simulink model "subwaycontrolsystem"  (R2012b)
settings: Solver=ode15s  StartTime=0.0  StopTime=2500  MaxStep=0.1  RelTol=1e-6
settings Model: Creator=fanghuixing  LastModifiedBy=fofo
settings SolverCC: MaxConsecutiveZCs=2000  ZeroCrossControl=DisableAll
settings DataIOCC: SignalLoggingSaveFormat=ModelDataLogs  InspectSignalLogs=on
settings OptimizationCC: EfficientMapNaN2IntZero=off
settings DebuggingCC: FcnCallInpInsideContextMsg=UseLocalSettings
settings HardwareCC: TargetIntDivRoundTo=Zero  TargetEndianess=LittleEndian  TargetHWDeviceType=MATLAB Host  ProdEqTarget=off
settings RTWCC: SystemTargetFile=accel.tlc  TemplateMakefile=accel_default_tmf  RTWVerbose=off  ProcessScript=accel_make_rtw_hook
settings CodeAppCC: MaxIdLength=128
settings STFCustomTargetCC: CodeReplacementLibrary=ANSI_C  ConcurrentExecutionCompliant=on  GeneratePreprocessorConditionals=Disable all  SystemTargetFile=accel.tlc

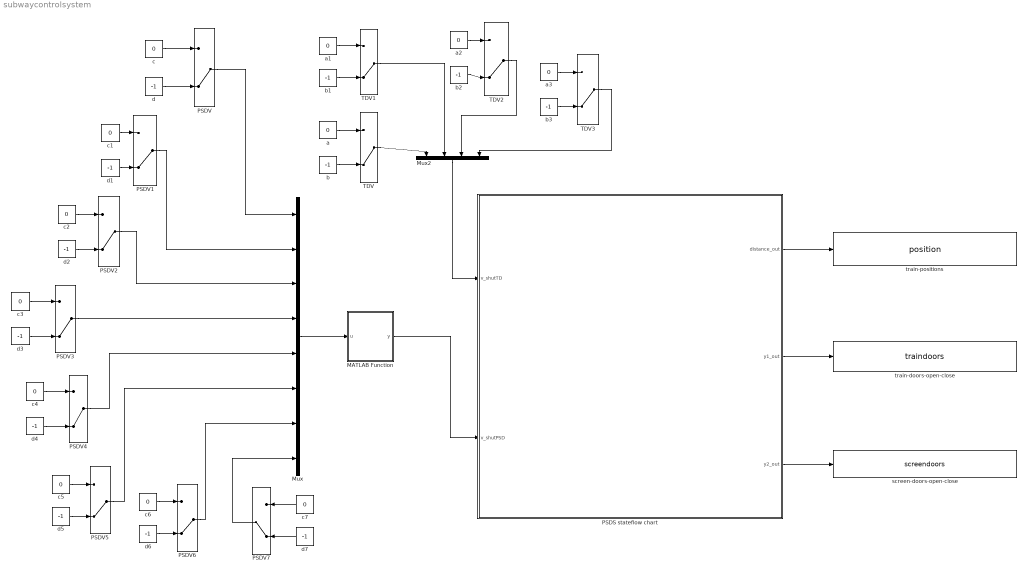
== system subwaycontrolsystem ==
  MATLAB Function : MATLAB Function  TreatAsAtomicUnit=on
  Mux : Mux  Inputs=8
  Mux2 : Mux
  PSDS stateflow chart : Stateflow chart  RequirementInfo="{}  %GIDa_87fe0a43_5411_4934_b3a9_58160d32c6a6"  TreatAsAtomicUnit=on
  PSDV{,1..7} (8 alike) : ManualSwitch  CurrentSetting=0
  TDV{,1..3} (4 alike) : ManualSwitch  CurrentSetting=0
  a{,1..3} (4 alike) : Constant  Value=0
  b{,1..3} (4 alike) : Constant  Value=-1
  c{,1..7} (8 alike) : Constant  Value=0
  "d   " : Constant  Value=-1
  d{1..7} (7 alike) : Constant  Value=-1
  screen-doors-open-close : ToWorkspace  VariableName=screendoors  SampleTime=-1  SaveFormat=Timeseries
  train-doors-open-close : ToWorkspace  VariableName=traindoors  SampleTime=-1  SaveFormat=Structure With Time
  train-positions : ToWorkspace  VariableName=position  SampleTime=-1  SaveFormat=Timeseries
  wires:
  a/1 -> TDV/1
  b/1 -> TDV/2
  TDV/1 -> Mux2/1
  c/1 -> PSDV/1
  "d   "/1 -> PSDV/2
  c1/1 -> PSDV1/1
  d1/1 -> PSDV1/2
  c2/1 -> PSDV2/1
  d2/1 -> PSDV2/2
  c3/1 -> PSDV3/1
  d3/1 -> PSDV3/2
  c4/1 -> PSDV4/1
  d4/1 -> PSDV4/2
  c5/1 -> PSDV5/1
  d5/1 -> PSDV5/2
  c6/1 -> PSDV6/1
  d6/1 -> PSDV6/2
  c7/1 -> PSDV7/1
  d7/1 -> PSDV7/2
  Mux2/1 -> PSDS stateflow chart/1(v_shutTD)
  a1/1 -> TDV1/1
  b1/1 -> TDV1/2
  TDV1/1 -> Mux2/2
  a2/1 -> TDV2/1
  b2/1 -> TDV2/2
  TDV2/1 -> Mux2/3
  a3/1 -> TDV3/1
  b3/1 -> TDV3/2
  TDV3/1 -> Mux2/4
  PSDV/1 -> Mux/1
  PSDV1/1 -> Mux/2
  PSDV2/1 -> Mux/3
  PSDV3/1 -> Mux/4
  PSDV4/1 -> Mux/5
  PSDV5/1 -> Mux/6
  Mux/1 -> MATLAB Function/1(u)
  PSDV6/1 -> Mux/7
  PSDV7/1 -> Mux/8
  MATLAB Function/1(y) -> PSDS stateflow chart/2(v_shutPSD)
  PSDS stateflow chart/2(y1_out) -> train-doors-open-close/1
  PSDS stateflow chart/3(y2_out) -> screen-doors-open-close/1
  PSDS stateflow chart/1(distance_out) -> train-positions/1

== stateflow chart subwaycontrolsystem/PSDS stateflow chart ==
  settings: updateMethod=CONTINUOUS
  state UrgentController [parallel]
    settings: executionOrder=14
    state tmp
      en:t=0;
      du:t_dot=0.5;
    state Delay
      en:t=0;
      du:t_dot=1;
    state D1
      en:t=0;
      du:t_dot=0.5;
    (default) -> Delay
    (junction 1294) -> UrgentController.tmp : {stopDecision(i);}
    UrgentController.tmp -> D1 : [t>=0]
        | {CalDistance(),
        | i=i+1;}
    Delay -> D1 : [t>=150]
        | {i=0;}
    D1 -> (junction 1294) [order 1] : [i!=N&&t>=0]
    D1 -> D1 [order 2] : [i==N&&t>=1]{i=0}
  state Controller1 [parallel]
    settings: executionOrder=16
    state about_to_close2
      en:z=0;
      du:z_dot=1;
    state start
      en:z=0;
      du:z_dot=1;
    state about_to_open2
      en:z=0;
      stop[i]=0;
      du:z_dot=1;
    state idle
      en:z=0;
      du:z_dot=1;
    state about_to_open1
      en:z=0;
      du:z_dot=1;
    state about_to_close1
      en:z=0;
      du:z_dot=1;
    state open1
      en:z=0;
      du:z_dot=1;
    state ring
      du:z_dot=1;
    Controller1.start -> Controller1.start [order 2] : [PSDClosed[stationid][side]==0]
    Controller1.about_to_close2 -> Controller1.about_to_close2 [order 1] : [in(Train1_door.closed)==0]
    (default) -> Controller1.idle
    Controller1.about_to_close1 -> Controller1.about_to_close2 : [z>=5]{closeTD[i]=1;}
    Controller1.about_to_close2 -> Controller1.start [order 2] : [z>=5]
        | {closePSD[stationid][side]=1;}
    Controller1.idle -> Controller1.about_to_open2 [order 1] : [stop[i]==1]
        | {i=1,stationid=Train1.j,
        | side=(dir[i]+1)/2}
    Controller1.start -> Controller1.idle [order 1] : [z>=5]{start[i]=1;}
    Controller1.idle -> Controller1.idle [order 2] : [z>=1&&stop[i]!=1]
        | {position[i]=Train1.distance}
    Controller1.about_to_open2 -> Controller1.about_to_open1 : [z>=5]{openPSD[stationid][side]=1;}
    Controller1.open1 -> Controller1.ring : [z>=10]
    Controller1.about_to_open1 -> Controller1.open1 : [z>=1]{openTD[i]=1;}
    Controller1.ring -> Controller1.about_to_close1 : [z>=20&&z<=30]
  state Train0 [parallel]
    settings: executionOrder=19
    state urgent_inc
      en:urstart[i]=0;
      du:
      distance_dot=dir[i]*v;
      v_dot=0.5;
      distance_out[i]=distance;
    state recover
      du:distance_dot=dir[i]*v;
      v_dot=-0.5;
      distance_out[i]=distance;
    state select
    state urgent_stop
      du:distance_dot=0;
      v_dot=0;distance_out[i]=distance;
      ex:maxv=sqrt(0.5*abs(S[j]-distance))
    state init
      du:time_dot=1;
    state near
      du:
      distance_dot=dir[i]*v;
      v_dot=acc;
      distance_out[i]=distance;
    state urgent_dec
      du:
      distance_dot=dir[i]*v;
      v_dot=-1.5;
      distance_out[i]=distance;
    state stop
      en:v=0;
    state tmp
    state stablerun
      du:
      distance_dot=dir[i]*v;
      v_dot=0;
      distance_out[i]=distance;
    state run
      du:distance_dot=dir[i]*v;
      v_dot=0.5;
      distance_out[i]=distance;
    state ChangeDirection
      du:time_dot=1;
    (default) -> Train0.init : {i=0,start[i]=0,stop[i]=0,
        | time=0,distance=0,
        | v=0,dir[i]=1;}
    Train0.urgent_inc -> Train0.recover [order 1] : [v>=maxv]
    Train0.select -> Train0.run [order 1] : [maxv>20]
    Train0.select -> Train0.urgent_inc [order 2] : [maxv<=20]
    Train0.urgent_stop -> Train0.select : [urstart[i]==1]
    Train0.recover -> (junction 1640) [order 1] : [urstop[i]==1]
    Train0.recover -> Train0.stop [order 2] : [abs(distance-S[j])<=1]
        | {stop[i]=1,v=0,start[i]=0;}
    Train0.urgent_inc -> (junction 1640) [order 2] : [urstop[i]==1]
    (junction 1640) -> Train0.urgent_dec
    Train0.urgent_dec -> Train0.urgent_stop : [v<=0.1]
        | {urstopped[i]=1;}
    Train0.init -> Train0.stop : [time>=Delay[i]]{stop[i]=1,j=0;}
    Train0.near -> Train0.stop [order 1] : [abs(distance-S[j])<=1]
        | {stop[i]=1,start[i]=0;}
    Train0.near -> Train0.urgent_dec [order 2] : [urstop[i]==1]
    Train0.stop -> Train0.tmp : [start[i]==1]
        | {stop[i]=0,time=0;}
    Train0.ChangeDirection -> Train0.stop : [time>=30]
        | {dir[i]=-dir[i],
        | stop[i]=1,
        | start[i]=0;}
    (junction 1641) -> Train0.near : {acc=-v^2*0.001}
    Train0.run -> Train0.urgent_dec [order 3] : [urstop[i]==1]
    Train0.stablerun -> Train0.urgent_dec [order 2] : [urstop[i]==1]
    Train0.tmp -> Train0.run [order 3] : [(dir[i]==1&&j<N-1)||(dir[i]==-1&&j>0)]
        | {j=j+dir[i];}
    Train0.tmp -> Train0.ChangeDirection [order 1] : [j==0&&dir[i]==-1]
    Train0.tmp -> Train0.ChangeDirection [order 2] : [j==N-1&&dir[i]==1]
    Train0.stablerun -> (junction 1641) [order 1] : [abs(distance-S[j])<=500]
    Train0.run -> (junction 1641) [order 1] : [abs(distance-S[j])<=500]
    Train0.run -> Train0.stablerun [order 2] : [v>=20]
  state Controller0 [parallel]
    settings: executionOrder=3
    state about_to_close2
      en:z=0;
      du:z_dot=1;
    state start
      en:z=0;
      du:z_dot=1;
    state about_to_open2
      en:z=0;
      stop[i]=0;
      du:z_dot=1;
    state idle
      en:z=0;
      du:z_dot=1;
    state about_to_open1
      en:z=0;
      du:z_dot=1;
    state about_to_close1
      en:z=0;
      du:z_dot=1;
    state open1
      en:z=0;
      du:z_dot=1;
    state ring
      du:z_dot=1;
    Controller0.start -> Controller0.start [order 2] : [PSDClosed[stationid][side]==0]
    Controller0.about_to_close2 -> Controller0.about_to_close2 [order 1] : [in(Train0_door.closed)==0]
    (default) -> Controller0.idle
    Controller0.about_to_close1 -> Controller0.about_to_close2 : [z>=5]{closeTD[i]=1;}
    Controller0.about_to_close2 -> Controller0.start [order 2] : [z>=5]
        | {closePSD[stationid][side]=1;}
    Controller0.idle -> Controller0.about_to_open2 [order 1] : [stop[i]==1]
        | {i=0,stationid=Train0.j,
        | side=(dir[i]+1)/2}
    Controller0.start -> Controller0.idle [order 1] : [z>=5]{start[i]=1;}
    Controller0.idle -> Controller0.idle [order 2] : [z>=1&&stop[i]!=1]
        | {position[i]=Train0.distance}
    Controller0.about_to_open2 -> Controller0.about_to_open1 : [z>=5]{openPSD[stationid][side]=1;}
    Controller0.open1 -> Controller0.ring : [z>=10]
    Controller0.about_to_open1 -> Controller0.open1 : [z>=1]{openTD[i]=1;}
    Controller0.ring -> Controller0.about_to_close1 : [z>=20&&z<=30]
  state Train0_door [parallel]
    settings: executionOrder=1
    state open
      en:y1=2;y1_out[0]=y1;
      du:y1_dot=0;
      y1_out[0]=y1;
    state part
      du:y1_dot=1;
      y1_out[0]=y1;
    state closed
      en:y1=0;y1_out[0]=y1;
      closeTD[0]=0;
      du:y1_dot=0;
    state shut
      du:y1_dot=v_shutTD[0];
      y1_out[0]=y1;
    Train0_door.part -> Train0_door.open : [y1>=2]
    Train0_door.closed -> Train0_door.part : [openTD[0]==1]/openTD[0]=0;
    Train0_door.open -> Train0_door.shut : [closeTD[0]==1]
    Train0_door.shut -> Train0_door.part [order 1] : [y1>0&&v_shutTD[0]==0]
    (default) -> Train0_door.closed
    Train0_door.shut -> Train0_door.closed [order 2] : [y1<=0]
  state Train1_door [parallel]
    settings: executionOrder=11
    state open
      en:y1=2;y1_out[1]=y1;
      du:y1_dot=0;
      y1_out[1]=y1;
    state part
      du:y1_dot=1;
      y1_out[1]=y1;
    state closed
      en:y1=0;y1_out[1]=y1;
      closeTD[1]=0;
      du:y1_dot=0;
    state shut
      du:y1_dot=v_shutTD[1];
      y1_out[1]=y1;
    Train1_door.part -> Train1_door.open : [y1>=2]
    Train1_door.closed -> Train1_door.part : [openTD[1]==1]/openTD[1]=0;
    Train1_door.open -> Train1_door.shut : [closeTD[1]==1]
    Train1_door.shut -> Train1_door.part [order 1] : [y1>0&&v_shutTD[1]==0]
    (default) -> Train1_door.closed
    Train1_door.shut -> Train1_door.closed [order 2] : [y1<=0]
  state Train1 [parallel]
    settings: executionOrder=20
    state urgent_inc
      en:urstart[i]=0;
      du:
      distance_dot=dir[i]*v;
      v_dot=0.5;
      distance_out[i]=distance;
    state recover
      du:distance_dot=dir[i]*v;
      v_dot=-0.5;
      distance_out[i]=distance;
    state select
    state urgent_stop
      du:distance_dot=0;
      v_dot=0;distance_out[i]=distance;
      ex:maxv=sqrt(0.5*abs(S[j]-distance))
    state init
      du:time_dot=1;
    state near
      du:
      distance_dot=dir[i]*v;
      v_dot=acc;
      distance_out[i]=distance;
    state urgent_dec
      du:
      distance_dot=dir[i]*v;
      v_dot=-1.5;
      distance_out[i]=distance;
    state stop
      en:v=0;
    state tmp
    state stablerun
      du:
      distance_dot=dir[i]*v;
      v_dot=0;
      distance_out[i]=distance;
    state run
      du:distance_dot=dir[i]*v;
      v_dot=0.5;
      distance_out[i]=distance;
    state ChangeDirection
      du:time_dot=1;
    (default) -> Train1.init : {i=1,start[i]=0,stop[i]=0,
        | time=0,distance=0,
        | v=0,dir[i]=1;}
    Train1.urgent_inc -> Train1.recover [order 1] : [v>=maxv]
    Train1.select -> Train1.run [order 1] : [maxv>20]
    Train1.select -> Train1.urgent_inc [order 2] : [maxv<=20]
    Train1.urgent_stop -> Train1.select : [urstart[i]==1]
    Train1.recover -> (junction 1686) [order 1] : [urstop[i]==1]
    Train1.recover -> Train1.stop [order 2] : [abs(distance-S[j])<=1]
        | {stop[i]=1,v=0,start[i]=0;}
    Train1.urgent_inc -> (junction 1686) [order 2] : [urstop[i]==1]
    (junction 1686) -> Train1.urgent_dec
    Train1.urgent_dec -> Train1.urgent_stop : [v<=0.1]
        | {urstopped[i]=1;}
    Train1.init -> Train1.stop : [time>=Delay[i]]{stop[i]=1,j=0;}
    Train1.near -> Train1.stop [order 1] : [abs(distance-S[j])<=1]
        | {stop[i]=1,start[i]=0;}
    Train1.near -> Train1.urgent_dec [order 2] : [urstop[i]==1]
    Train1.stop -> Train1.tmp : [start[i]==1]
        | {stop[i]=0,time=0;}
    Train1.ChangeDirection -> Train1.stop : [time>=30]
        | {dir[i]=-dir[i],
        | stop[i]=1,
        | start[i]=0;}
    (junction 1687) -> Train1.near : {acc=-v^2*0.001}
    Train1.run -> Train1.urgent_dec [order 3] : [urstop[i]==1]
    Train1.stablerun -> Train1.urgent_dec [order 2] : [urstop[i]==1]
    Train1.tmp -> Train1.run [order 3] : [(dir[i]==1&&j<N-1)||(dir[i]==-1&&j>0)]
        | {j=j+dir[i];}
    Train1.tmp -> Train1.ChangeDirection [order 1] : [j==0&&dir[i]==-1]
    Train1.tmp -> Train1.ChangeDirection [order 2] : [j==N-1&&dir[i]==1]
    Train1.stablerun -> (junction 1687) [order 1] : [abs(distance-S[j])<=500]
    Train1.run -> (junction 1687) [order 1] : [abs(distance-S[j])<=500]
    Train1.run -> Train1.stablerun [order 2] : [v>=20]
  state Controller3 [parallel]
    settings: executionOrder=18
    state about_to_close2
      en:z=0;
      du:z_dot=1;
    state start
      en:z=0;
      du:z_dot=1;
    state about_to_open2
      en:z=0;
      stop[i]=0;
      du:z_dot=1;
    state idle
      en:z=0;
      du:z_dot=1;
    state about_to_open1
      en:z=0;
      du:z_dot=1;
    state about_to_close1
      en:z=0;
      du:z_dot=1;
    state open1
      en:z=0;
      du:z_dot=1;
    state ring
      du:z_dot=1;
    Controller3.start -> Controller3.start [order 2] : [PSDClosed[stationid][side]==0]
    Controller3.about_to_close2 -> Controller3.about_to_close2 [order 1] : [in(Train3_door.closed)==0]
    (default) -> Controller3.idle
    Controller3.about_to_close1 -> Controller3.about_to_close2 : [z>=5]{closeTD[i]=1;}
    Controller3.about_to_close2 -> Controller3.start [order 2] : [z>=5]
        | {closePSD[stationid][side]=1;}
    Controller3.idle -> Controller3.about_to_open2 [order 1] : [stop[i]==1]
        | {i=3,stationid=Train3.j,
        | side=(dir[i]+1)/2}
    Controller3.start -> Controller3.idle [order 1] : [z>=5]{start[i]=1;}
    Controller3.idle -> Controller3.idle [order 2] : [z>=1&&stop[i]!=1]
        | {position[i]=Train3.distance}
    Controller3.about_to_open2 -> Controller3.about_to_open1 : [z>=5]{openPSD[stationid][side]=1;}
    Controller3.open1 -> Controller3.ring : [z>=10]
    Controller3.about_to_open1 -> Controller3.open1 : [z>=1]{openTD[i]=1;}
    Controller3.ring -> Controller3.about_to_close1 : [z>=20&&z<=30]
  state Controller2 [parallel]
    settings: executionOrder=17
    state about_to_close2
      en:z=0;
      du:z_dot=1;
    state start
      en:z=0;
      du:z_dot=1;
    state about_to_open2
      en:z=0;
      stop[i]=0;
      du:z_dot=1;
    state idle
      en:z=0;
      du:z_dot=1;
    state about_to_open1
      en:z=0;
      du:z_dot=1;
    state about_to_close1
      en:z=0;
      du:z_dot=1;
    state open1
      en:z=0;
      du:z_dot=1;
    state ring
      du:z_dot=1;
    Controller2.start -> Controller2.start [order 2] : [PSDClosed[stationid][side]==0]
    Controller2.about_to_close2 -> Controller2.about_to_close2 [order 1] : [in(Train2_door.closed)==0]
    (default) -> Controller2.idle
    Controller2.about_to_close1 -> Controller2.about_to_close2 : [z>=5]{closeTD[i]=1;}
    Controller2.about_to_close2 -> Controller2.start [order 2] : [z>=5]
        | {closePSD[stationid][side]=1;}
    Controller2.idle -> Controller2.about_to_open2 [order 1] : [stop[i]==1]
        | {i=2,stationid=Train2.j,
        | side=(dir[i]+1)/2}
    Controller2.start -> Controller2.idle [order 1] : [z>=5]{start[i]=1;}
    Controller2.idle -> Controller2.idle [order 2] : [z>=1&&stop[i]!=1]
        | {position[i]=Train2.distance}
    Controller2.about_to_open2 -> Controller2.about_to_open1 : [z>=5]{openPSD[stationid][side]=1;}
    Controller2.open1 -> Controller2.ring : [z>=10]
    Controller2.about_to_open1 -> Controller2.open1 : [z>=1]{openTD[i]=1;}
    Controller2.ring -> Controller2.about_to_close1 : [z>=20&&z<=30]
  state Train2 [parallel]
    settings: executionOrder=21
    state urgent_inc
      en:urstart[i]=0;
      du:
      distance_dot=dir[i]*v;
      v_dot=0.5;
      distance_out[i]=distance;
    state recover
      du:distance_dot=dir[i]*v;
      v_dot=-0.5;
      distance_out[i]=distance;
    state select
    state urgent_stop
      du:distance_dot=0;
      v_dot=0;distance_out[i]=distance;
      ex:maxv=sqrt(0.5*abs(S[j]-distance))
    state init
      du:time_dot=1;
    state near
      du:
      distance_dot=dir[i]*v;
      v_dot=acc;
      distance_out[i]=distance;
    state urgent_dec
      du:
      distance_dot=dir[i]*v;
      v_dot=-1.5;
      distance_out[i]=distance;
    state stop
      en:v=0;
    state tmp
    state stablerun
      du:
      distance_dot=dir[i]*v;
      v_dot=0;
      distance_out[i]=distance;
    state run
      du:distance_dot=dir[i]*v;
      v_dot=0.5;
      distance_out[i]=distance;
    state ChangeDirection
      du:time_dot=1;
    (default) -> Train2.init : {i=2,start[i]=0,stop[i]=0,
        | time=0,distance=0,
        | v=0,dir[i]=1;}
    Train2.urgent_inc -> Train2.recover [order 1] : [v>=maxv]
    Train2.select -> Train2.run [order 1] : [maxv>20]
    Train2.select -> Train2.urgent_inc [order 2] : [maxv<=20]
    Train2.urgent_stop -> Train2.select : [urstart[i]==1]
    Train2.recover -> (junction 1732) [order 1] : [urstop[i]==1]
    Train2.recover -> Train2.stop [order 2] : [abs(distance-S[j])<=1]
        | {stop[i]=1,v=0,start[i]=0;}
    Train2.urgent_inc -> (junction 1732) [order 2] : [urstop[i]==1]
    (junction 1732) -> Train2.urgent_dec
    Train2.urgent_dec -> Train2.urgent_stop : [v<=0.1]
        | {urstopped[i]=1;}
    Train2.init -> Train2.stop : [time>=Delay[i]]{stop[i]=1,j=0;}
    Train2.near -> Train2.stop [order 1] : [abs(distance-S[j])<=1]
        | {stop[i]=1,start[i]=0;}
    Train2.near -> Train2.urgent_dec [order 2] : [urstop[i]==1]
    Train2.stop -> Train2.tmp : [start[i]==1]
        | {stop[i]=0,time=0;}
    Train2.ChangeDirection -> Train2.stop : [time>=30]
        | {dir[i]=-dir[i],
        | stop[i]=1,
        | start[i]=0;}
    (junction 1733) -> Train2.near : {acc=-v^2*0.001}
    Train2.run -> Train2.urgent_dec [order 3] : [urstop[i]==1]
    Train2.stablerun -> Train2.urgent_dec [order 2] : [urstop[i]==1]
    Train2.tmp -> Train2.run [order 3] : [(dir[i]==1&&j<N-1)||(dir[i]==-1&&j>0)]
        | {j=j+dir[i];}
    Train2.tmp -> Train2.ChangeDirection [order 1] : [j==0&&dir[i]==-1]
    Train2.tmp -> Train2.ChangeDirection [order 2] : [j==N-1&&dir[i]==1]
    Train2.stablerun -> (junction 1733) [order 1] : [abs(distance-S[j])<=500]
    Train2.run -> (junction 1733) [order 1] : [abs(distance-S[j])<=500]
    Train2.run -> Train2.stablerun [order 2] : [v>=20]
  state Train2_door [parallel]
    settings: executionOrder=12
    state open
      en:y1=2;y1_out[2]=y1;
      du:y1_dot=0;
      y1_out[2]=y1;
    state part
      du:y1_dot=1;
      y1_out[2]=y1;
    state closed
      en:y1=0;y1_out[2]=y1;
      closeTD[2]=0;
      du:y1_dot=0;
    state shut
      du:y1_dot=v_shutTD[2];
      y1_out[2]=y1;
    Train2_door.part -> Train2_door.open : [y1>=2]
    Train2_door.closed -> Train2_door.part : [openTD[2]==1]/openTD[2]=0;
    Train2_door.open -> Train2_door.shut : [closeTD[2]==1]
    Train2_door.shut -> Train2_door.part [order 1] : [y1>0&&v_shutTD[2]==0]
    (default) -> Train2_door.closed
    Train2_door.shut -> Train2_door.closed [order 2] : [y1<=0]
  state Train3 [parallel]
    settings: executionOrder=15
    state urgent_inc
      en:urstart[i]=0;
      du:
      distance_dot=dir[i]*v;
      v_dot=0.5;
      distance_out[i]=distance;
    state recover
      du:distance_dot=dir[i]*v;
      v_dot=-0.5;
      distance_out[i]=distance;
    state select
    state urgent_stop
      du:distance_dot=0;
      v_dot=0;distance_out[i]=distance;
      ex:maxv=sqrt(0.5*abs(S[j]-distance))
    state init
      du:time_dot=1;
    state near
      du:
      distance_dot=dir[i]*v;
      v_dot=acc;
      distance_out[i]=distance;
    state urgent_dec
      du:
      distance_dot=dir[i]*v;
      v_dot=-1.5;
      distance_out[i]=distance;
    state stop
      en:v=0;
    state tmp
    state stablerun
      du:
      distance_dot=dir[i]*v;
      v_dot=0;
      distance_out[i]=distance;
    state run
      du:distance_dot=dir[i]*v;
      v_dot=0.5;
      distance_out[i]=distance;
    state ChangeDirection
      du:time_dot=1;
    (default) -> Train3.init : {i=3,start[i]=0,stop[i]=0,
        | time=0,distance=0,
        | v=0,dir[i]=1;}
    Train3.urgent_inc -> Train3.recover [order 1] : [v>=maxv]
    Train3.select -> Train3.run [order 1] : [maxv>20]
    Train3.select -> Train3.urgent_inc [order 2] : [maxv<=20]
    Train3.urgent_stop -> Train3.select : [urstart[i]==1]
    Train3.recover -> (junction 1422) [order 1] : [urstop[i]==1]
    Train3.recover -> Train3.stop [order 2] : [abs(distance-S[j])<=1]
        | {stop[i]=1,v=0,start[i]=0;}
    Train3.urgent_inc -> (junction 1422) [order 2] : [urstop[i]==1]
    (junction 1422) -> Train3.urgent_dec
    Train3.urgent_dec -> Train3.urgent_stop : [v<=0.1]
        | {urstopped[i]=1;}
    Train3.init -> Train3.stop : [time>=Delay[i]]{stop[i]=1,j=0;}
    Train3.near -> Train3.stop [order 1] : [abs(distance-S[j])<=1]
        | {stop[i]=1,start[i]=0;}
    Train3.near -> Train3.urgent_dec [order 2] : [urstop[i]==1]
    Train3.stop -> Train3.tmp : [start[i]==1]
        | {stop[i]=0,time=0;}
    Train3.ChangeDirection -> Train3.stop : [time>=30]
        | {dir[i]=-dir[i],
        | stop[i]=1,
        | start[i]=0;}
    (junction 1423) -> Train3.near : {acc=-v^2*0.001}
    Train3.run -> Train3.urgent_dec [order 3] : [urstop[i]==1]
    Train3.stablerun -> Train3.urgent_dec [order 2] : [urstop[i]==1]
    Train3.tmp -> Train3.run [order 3] : [(dir[i]==1&&j<N-1)||(dir[i]==-1&&j>0)]
        | {j=j+dir[i];}
    Train3.tmp -> Train3.ChangeDirection [order 1] : [j==0&&dir[i]==-1]
    Train3.tmp -> Train3.ChangeDirection [order 2] : [j==N-1&&dir[i]==1]
    Train3.stablerun -> (junction 1423) [order 1] : [abs(distance-S[j])<=500]
    Train3.run -> (junction 1423) [order 1] : [abs(distance-S[j])<=500]
    Train3.run -> Train3.stablerun [order 2] : [v>=20]
  state Train3_door [parallel]
    settings: executionOrder=13
    state open
      en:y1=2;y1_out[3]=y1;
      du:y1_dot=0;
      y1_out[3]=y1;
    state part
      du:y1_dot=1;
      y1_out[3]=y1;
    state closed
      en:y1=0;y1_out[3]=y1;
      closeTD[3]=0;
      du:y1_dot=0;
    state shut
      du:y1_dot=v_shutTD[3];
      y1_out[3]=y1;
    Train3_door.part -> Train3_door.open : [y1>=2]
    Train3_door.closed -> Train3_door.part : [openTD[3]==1]/openTD[3]=0;
    Train3_door.open -> Train3_door.shut : [closeTD[3]==1]
    Train3_door.shut -> Train3_door.part [order 1] : [y1>0&&v_shutTD[3]==0]
    (default) -> Train3_door.closed
    Train3_door.shut -> Train3_door.closed [order 2] : [y1<=0]
  state Screen_door10 [parallel]
    settings: executionOrder=5
    state part
      du:y2_dot=1;
      y2_out[1][0]=y2;
    state open
      en:y2=2;y2_out[1][0]=y2;
      du:y2_dot=0;
      y2_out[1][0]=y2;
    state shut
      du:y2_dot=v_shutPSD[1][0];
      y2_out[1][0]=y2;
    state closed
      en:y2=0;y2_out[1][0]=y2;
      closePSD[1][0]=0;
      du:y2_dot=0;
    Screen_door10.part -> Screen_door10.open : [y2>=2]
    Screen_door10.closed -> Screen_door10.part : [openPSD[1][0]==1]{PSDClosed[1][0]=0}
        | /openPSD[1][0]=0;
    Screen_door10.shut -> Screen_door10.part [order 2] : [y2>0&&v_shutPSD[1][0]==0]
    Screen_door10.open -> Screen_door10.shut : [closePSD[1][0]==1]
    (default) -> Screen_door10.closed : {PSDClosed[1][0]=1}
    Screen_door10.shut -> Screen_door10.closed [order 1] : [y2<=0]{PSDClosed[1][0]=1}
  state Screen_door11 [parallel]
    settings: executionOrder=6
    state part
      du:y2_dot=1;
      y2_out[1][1]=y2;
    state open
      en:y2=2;y2_out[1][1]=y2;
      du:y2_dot=0;
      y2_out[1][1]=y2;
    state shut
      du:y2_dot=v_shutPSD[1][1];
      y2_out[1][1]=y2;
    state closed
      en:y2=0;y2_out[1][1]=y2;
      closePSD[1][1]=0;
      du:y2_dot=0;
    Screen_door11.part -> Screen_door11.open : [y2>=2]
    Screen_door11.closed -> Screen_door11.part : [openPSD[1][1]==1]{PSDClosed[1][1]=0}
        | /openPSD[1][1]=0;
    Screen_door11.shut -> Screen_door11.part [order 2] : [y2>0&&v_shutPSD[1][1]==0]
    Screen_door11.open -> Screen_door11.shut : [closePSD[1][1]==1]
    (default) -> Screen_door11.closed : {PSDClosed[1][1]=1}
    Screen_door11.shut -> Screen_door11.closed [order 1] : [y2<=0]{PSDClosed[1][1]=1}
  state Screen_door01 [parallel]
    settings: executionOrder=4
    state part
      du:y2_dot=1;
      y2_out[0][1]=y2;
    state open
      en:y2=2;y2_out[0][1]=y2;
      du:y2_dot=0;
      y2_out[0][1]=y2;
    state shut
      du:y2_dot=v_shutPSD[0][1];
      y2_out[0][1]=y2;
    state closed
      en:y2=0;y2_out[0][1]=y2;
      closePSD[0][1]=0;
      du:y2_dot=0;
    Screen_door01.part -> Screen_door01.open : [y2>=2]
    Screen_door01.closed -> Screen_door01.part : [openPSD[0][1]==1]{PSDClosed[0][1]=0}
        | /openPSD[0][1]=0;
    Screen_door01.shut -> Screen_door01.part [order 2] : [y2>0&&v_shutPSD[0][1]==0]
    Screen_door01.open -> Screen_door01.shut : [closePSD[0][1]==1]
    (default) -> Screen_door01.closed : {PSDClosed[0][1]=1}
    Screen_door01.shut -> Screen_door01.closed [order 1] : [y2<=0]{PSDClosed[0][1]=1}
  state Screen_door00 [parallel]
    settings: executionOrder=2
    state part
      du:y2_dot=1;
      y2_out[0][0]=y2;
    state open
      en:y2=2;y2_out[0][0]=y2;
      du:y2_dot=0;
      y2_out[0][0]=y2;
    state shut
      du:y2_dot=v_shutPSD[0][0];
      y2_out[0][0]=y2;
    state closed
      en:y2=0;y2_out[0][0]=y2;
      closePSD[0][0]=0;
      du:y2_dot=0;
    Screen_door00.part -> Screen_door00.open : [y2>=2]
    Screen_door00.closed -> Screen_door00.part : [openPSD[0][0]==1]{PSDClosed[0][0]=0}
        | /openPSD[0][0]=0;
    Screen_door00.shut -> Screen_door00.part [order 2] : [y2>0&&v_shutPSD[0][0]==0]
    Screen_door00.open -> Screen_door00.shut : [closePSD[0][0]==1]
    (default) -> Screen_door00.closed : {PSDClosed[0][0]=1}
    Screen_door00.shut -> Screen_door00.closed [order 1] : [y2<=0]{PSDClosed[0][0]=1}
  state Screen_door30 [parallel]
    settings: executionOrder=9
    state part
      du:y2_dot=1;
      y2_out[3][0]=y2;
    state open
      en:y2=2;y2_out[3][0]=y2;
      du:y2_dot=0;
      y2_out[3][0]=y2;
    state shut
      du:y2_dot=v_shutPSD[3][0];
      y2_out[3][0]=y2;
    state closed
      en:y2=0;y2_out=y2;
      closePSD[3][0]=0;
      du:y2_dot=0;
    Screen_door30.part -> Screen_door30.open : [y2>=2]
    Screen_door30.closed -> Screen_door30.part : [openPSD[3][0]==1]{PSDClosed[3][0]=0}
        | /openPSD[3][0]=0;
    Screen_door30.shut -> Screen_door30.part [order 2] : [y2>0&&v_shutPSD[3][0]==0]
    Screen_door30.open -> Screen_door30.shut : [closePSD[3][0]==1]
    (default) -> Screen_door30.closed : {PSDClosed[3][0]=1}
    Screen_door30.shut -> Screen_door30.closed [order 1] : [y2<=0]{PSDClosed[3][0]=1}
  state Screen_door31 [parallel]
    settings: executionOrder=10
    state part
      du:y2_dot=1;
      y2_out[3][1]=y2;
    state open
      en:y2=2;y2_out[3][1]=y2;
      du:y2_dot=0;
      y2_out[3][1]=y2;
    state shut
      du:y2_dot=v_shutPSD[3][1];
      y2_out[3][1]=y2;
    state closed
      en:y2=0;y2_out[3][1]=y2;
      closePSD[3][1]=0;
      du:y2_dot=0;
    Screen_door31.part -> Screen_door31.open : [y2>=2]
    Screen_door31.closed -> Screen_door31.part : [openPSD[3][1]==1]{PSDClosed[3][1]=0}
        | /openPSD[3][1]=0;
    Screen_door31.shut -> Screen_door31.part [order 2] : [y2>0&&v_shutPSD[3][1]==0]
    Screen_door31.open -> Screen_door31.shut : [closePSD[3][1]==1]
    (default) -> Screen_door31.closed : {PSDClosed[3][1]=1}
    Screen_door31.shut -> Screen_door31.closed [order 1] : [y2<=0]{PSDClosed[3][1]=1}
  state Screen_door21 [parallel]
    settings: executionOrder=8
    state part
      du:y2_dot=1;
      y2_out[2][1]=y2;
    state open
      en:y2=2;y2_out[2][1]=y2;
      du:y2_dot=0;
      y2_out[2][1]=y2;
    state shut
      du:y2_dot=v_shutPSD[2][1];
      y2_out[2][1]=y2;
    state closed
      en:y2=0;y2_out[2][1]=y2;
      closePSD[2][1]=0;
      du:y2_dot=0;
    Screen_door21.part -> Screen_door21.open : [y2>=2]
    Screen_door21.closed -> Screen_door21.part : [openPSD[2][1]==1]{PSDClosed[2][1]=0}
        | /openPSD[2][1]=0;
    Screen_door21.shut -> Screen_door21.part [order 2] : [y2>0&&v_shutPSD[2][1]==0]
    Screen_door21.open -> Screen_door21.shut : [closePSD[2][1]==1]
    (default) -> Screen_door21.closed : {PSDClosed[2][1]=1}
    Screen_door21.shut -> Screen_door21.closed [order 1] : [y2<=0]{PSDClosed[2][1]=1}
  state Screen_door20 [parallel]
    settings: executionOrder=7
    state part
      du:y2_dot=1;
      y2_out[2][0]=y2;
    state open
      en:y2=2;y2_out[2][0]=y2;
      du:y2_dot=0;
      y2_out[2][0]=y2;
    state shut
      du:y2_dot=v_shutPSD[2][0];
      y2_out[2][0]=y2;
    state closed
      en:y2=0;y2_out[2][0]=y2;
      closePSD[2][0]=0;
      du:y2_dot=0;
    Screen_door20.part -> Screen_door20.open : [y2>=2]
    Screen_door20.closed -> Screen_door20.part : [openPSD[2][0]==1]{PSDClosed[2][0]=0}
        | /openPSD[2][0]=0;
    Screen_door20.shut -> Screen_door20.part [order 2] : [y2>0&&v_shutPSD[2][0]==0]
    Screen_door20.open -> Screen_door20.shut : [closePSD[2][0]==1]
    (default) -> Screen_door20.closed : {PSDClosed[2][0]=1}
    Screen_door20.shut -> Screen_door20.closed [order 1] : [y2<=0]{PSDClosed[2][0]=1}
  data: a function_input double; t local double; i local int32; RelevantIndex local int32 size=[1 4] =[-1 -1 -1 -1]; tdis local int32; dis local int32; z local double; stationid local double; side local double; i local int32 =1; v local double; j local double; maxv local double; time local double; i local int32; distance local double; acc local double; z local double; stationid local double; side local double; i local int32 =0; y1 local double; y1 local double; v local double; j local double; maxv local double; time local double; i local int32; distance local double; acc local double; z local double; stationid local double; side local double; i local int32 =3; z local double; stationid local double; side local double; i local int32 =2; v local double; j local double; maxv local double; time local double; i local int32; distance local double; acc local double; y1 local double; v local double; j local double; maxv local double; time local double; i local int32; distance local double; acc local double; y1 local double; y2 local double; y2 local double; y2 local double; y2 local double; y2 local double; y2 local double; y2 local double; y2 local double; v_shutTD input size=[4 1]; v_shutPSD input size=[4 2]; start local double size=[4 1]; stop local double size=[1 4] =[0 0 0 0]; openPSD local double size=[4 2]; closePSD local double size=[4 2]; distance_out output double size=[4 1]; Delay local double size=[1 4] =[0 50 100 150]; openTD local double size=[4 1]; closeTD local double size=[4 1]; S local double size=[1 4] =[0 2284 3292 9097]; urstart local double size=[4 1]; urstop local double size=[4 1]; N local int32 =4; y1_out output double size=[4 1]; y2_out output double size=[4 2]; urstopped local double size=[4 1]; dir local int32 size=[4 1]; position local double size=[4 1]; PSDClosed local double size=[4 2]
  data t settings: updateMethod=SF_CONTINUOUS_TIME_DATA
  data z settings: updateMethod=SF_CONTINUOUS_TIME_DATA
  data v settings: updateMethod=SF_CONTINUOUS_TIME_DATA
  data time settings: updateMethod=SF_CONTINUOUS_TIME_DATA
  data distance settings: updateMethod=SF_CONTINUOUS_TIME_DATA
  data z settings: updateMethod=SF_CONTINUOUS_TIME_DATA
  data y1 settings: updateMethod=SF_CONTINUOUS_TIME_DATA
  data y1 settings: updateMethod=SF_CONTINUOUS_TIME_DATA
  data v settings: updateMethod=SF_CONTINUOUS_TIME_DATA
  data time settings: updateMethod=SF_CONTINUOUS_TIME_DATA
  data distance settings: updateMethod=SF_CONTINUOUS_TIME_DATA
  data z settings: updateMethod=SF_CONTINUOUS_TIME_DATA
  data z settings: updateMethod=SF_CONTINUOUS_TIME_DATA
  data v settings: updateMethod=SF_CONTINUOUS_TIME_DATA
  data time settings: updateMethod=SF_CONTINUOUS_TIME_DATA
  data distance settings: updateMethod=SF_CONTINUOUS_TIME_DATA
  data y1 settings: updateMethod=SF_CONTINUOUS_TIME_DATA
  data v settings: updateMethod=SF_CONTINUOUS_TIME_DATA
  data time settings: updateMethod=SF_CONTINUOUS_TIME_DATA
  data distance settings: updateMethod=SF_CONTINUOUS_TIME_DATA
  data y1 settings: updateMethod=SF_CONTINUOUS_TIME_DATA
  data y2 settings: updateMethod=SF_CONTINUOUS_TIME_DATA
  data y2 settings: updateMethod=SF_CONTINUOUS_TIME_DATA
  data y2 settings: updateMethod=SF_CONTINUOUS_TIME_DATA
  data y2 settings: updateMethod=SF_CONTINUOUS_TIME_DATA
  data y2 settings: updateMethod=SF_CONTINUOUS_TIME_DATA
  data y2 settings: updateMethod=SF_CONTINUOUS_TIME_DATA
  data y2 settings: updateMethod=SF_CONTINUOUS_TIME_DATA
  data y2 settings: updateMethod=SF_CONTINUOUS_TIME_DATA
  function CalDistance:
    | function CalDistance()
    | 
    | for index = 1:4
    |     si=index;
    |     sj=RelevantIndex(index);
    |     if sj~=-1 && urstopped(si)==1
    |         urstop(si)=0;
    |         if abs(position(sj)-position(si))>300 || dir(si)~=dir(sj)
    |             urstart(si)=1;
    |             urstopped(si)=0;
    |         end
    |     end
    | end
  function stopDecision(a):
    | function stopDecision(a)
    | 
    | dis=int32(10000);
    | needstop=0;
    | 
    | for index=0:N-1
    |     if a~= index && dir(a+1)==dir(index+1)
    |             tdis=dir(a+1)*(position(index+1)-position(a+1));
    |             if tdis<=300 && tdis>0
    |                 if tdis<dis
    |                         dis=tdis
    |                         RelevantIndex(a+1)=index+1;
    |                         needstop=1;                    
    |                 end
    |             end           
    |     end
    | end
    | 
    | if needstop==1
    |     urstop(a+1) = 1;
    | end

== matlab function subwaycontrolsystem/MATLAB Function ==
  data: u input; y output
function y = fcn(u)
%#codegen
y=zeros(4,2);
j=1;
k=1;
for i=1:8
    y(j,k)=u(i);
    if k==2
        k=1;
        j=j+1;
    else
        k=k+1;
    end
end
